simulink model "prestudio55"  (R2018b)
settings: Solver=ode45  StartTime=0.  StopTime=20  FixedStep=0.2  MaxStep=0.05  RelTol=1e-8  AbsTol=1e-8  EnableMultiTasking=on
settings Model: ExtModeTrigMode=oneshot  ExtModeArmWhenConnect=off  Creator=LEVIENKL  LastModifiedBy=Heidi Reed
settings SolverCC: AutoScaleAbsTol=off
settings DataIOCC: SaveFormat=Array  SignalLoggingSaveFormat=ModelDataLogs  SaveOutput=off  SaveTime=off  SignalLoggingName=sigsOut
settings OptimizationCC: BlockReduction=off  BooleanDataType=off  ExpressionDepthLimit=2147483647  InitFltsAndDblsToZero=on  LifeSpan=inf
settings DebuggingCC: SaveWithParameterizedLinksMsg=none  UnderspecifiedInitializationDetection=Classic  MergeDetectMultiDrivingBlocksExec=none  SignalResolutionControl=TryResolveAllWithWarning  MultiTaskDSMMsg=warning  MultiTaskCondExecSysMsg=none  FcnCallInpInsideContextMsg=warning  AllowSymbolicDim=off  StateNameClashWarn=warning  SFUnexpectedBacktrackingDiag=warning  SFNoUnconditionalDefaultTransitionDiag=warning  SFExecutionAtInitializationDiag=none
settings HardwareCC: ProdBitPerPointer=32  ProdBitPerSizeT=32  ProdBitPerPtrDiffT=32  ProdLargestAtomicFloat=None  ProdIntDivRoundTo=Undefined  ProdEndianess=Unspecified  ProdWordSize=32  ProdHWDeviceType=32-bit Generic  TargetUnknown=on
settings ModelReferenceCC: PropagateSignalLabelsOutOfModel=off
settings SFSimCC: SimUseLocalCustomCode=off
settings RTWCC: RTWUseLocalCustomCode=off
settings CodeAppCC: StateflowObjectComments=on
settings GRTTargetCC: TargetFcnLib=ansi_tfl_tmw.mat  TargetLangStandard=C89/C90 (ANSI)  CombineOutputUpdateFcns=off  GRTInterface=on
settings ConfigComp: CovMetricSettings=dw  CovHtmlReporting=on  CovSaveCumulativeToWorkspaceVar=on  CovSaveSingleToWorkspaceVar=on  CovExternalEMLEnable=off  CovSFcnEnable=off

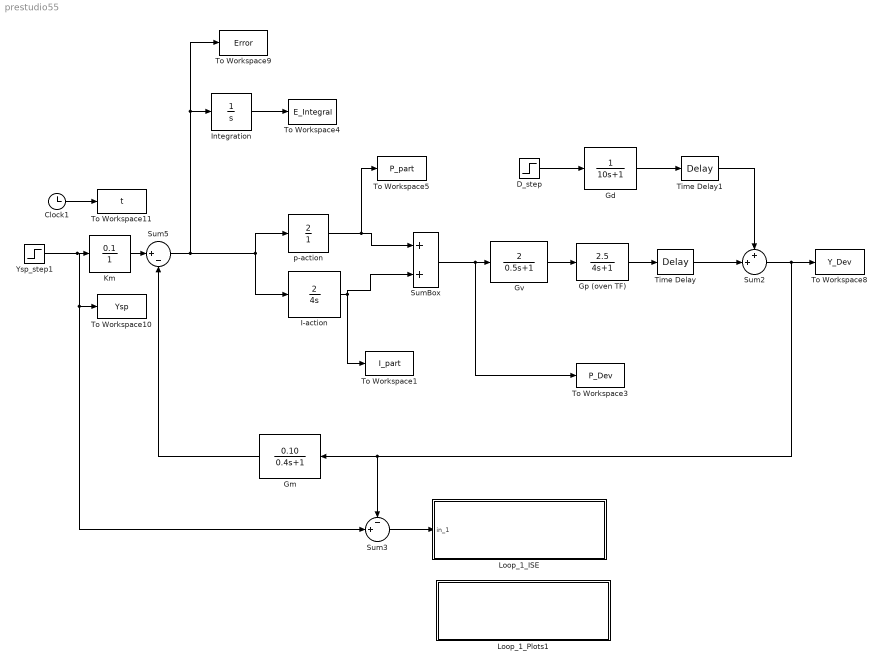
== system prestudio55 ==
  Clock1 : Clock
  D_step : Step  Time=0  After=0  SampleTime=0
      settings: AttributesFormatString=%<Before> to %<After>\nat %<Time>
  Gd : TransferFcn  Denominator=[10 1]
  Gm : TransferFcn  Numerator=[0.10]  Denominator=[0.4 1]
  Gp (oven TF) : TransferFcn  Numerator=[2.5]  Denominator=[4 1]
  Gv : TransferFcn  Numerator=[2]  Denominator=[0.5 1]
  "I-action " : TransferFcn  Numerator=[2]  Denominator=[4 0]
  "Integration " : TransferFcn  Denominator=[1 0]
  "Km " : TransferFcn  Numerator=[0.1]  Denominator=[0 1]
  Loop_1_ISE : Subsystem  mask(Integral Squarred Evaluation - Loop 1){}
      settings: OpenFcn=ISE1
      mask Help: This block calculates and plots loop #1 ISE.
      mask Display: disp('After Loop 1 Simulation:\n Double Click for ISE evaluation\n (uses ISE1.p)')
  Loop_1_Plots1 : Subsystem  mask(Y,U,E Plots - Loop 1){}
      settings: OpenFcn=YPEplots
      mask Help: This block loop #1 Y,U,Error in 3x1 Figure Window.
      mask Display: disp('After Loop 1 Simulation:\n Double Click for Y, P, Error Plots\n (uses YPEplots.p)')
  Sum2 : Sum  Inputs=++|  InputSameDT=on  SaturateOnIntegerOverflow=on  OutDataTypeStr=Inherit: Same as first input
  Sum3 : Sum  Inputs=-+|  InputSameDT=on  SaturateOnIntegerOverflow=on  OutDataTypeStr=Inherit: Same as first input
  Sum5 : Sum  Inputs=|+-  InputSameDT=on  SaturateOnIntegerOverflow=on  OutDataTypeStr=Inherit: Same as first input
  SumBox : Sum
  Time Delay : TransportDelay  DelayTime=0
      settings: AttributesFormatString=Delay=%<DelayTime>
  Time Delay1 : TransportDelay  DelayTime=0
      settings: AttributesFormatString=Delay=%<DelayTime>
  To Workspace1 : ToWorkspace  VariableName=I_part  SampleTime=-1
  To Workspace10 : ToWorkspace  VariableName=Ysp  SampleTime=-1
  To Workspace11 : ToWorkspace  VariableName=t  SampleTime=-1
  To Workspace3 : ToWorkspace  VariableName=P_Dev  SampleTime=-1
  To Workspace4 : ToWorkspace  VariableName=E_Integral  SampleTime=-1
  To Workspace5 : ToWorkspace  VariableName=P_part  SampleTime=-1
  To Workspace8 : ToWorkspace  VariableName=Y_Dev  SampleTime=-1
  To Workspace9 : ToWorkspace  VariableName=Error  SampleTime=-1
  Ysp_step1 : Step  Time=2  After=5  SampleTime=0
      settings: AttributesFormatString=%<Before> to %<After>\nat %<Time>
  "p-action " : TransferFcn  Numerator=[2]  Denominator=[0 1]
  wires:
  Ysp_step1/1 -> "Km "/1, Sum3/2, To Workspace10/1
  Sum5/1 -> "p-action "/1, "I-action "/1, "Integration "/1, To Workspace9/1
  "I-action "/1 -> SumBox/2, To Workspace1/1
  "p-action "/1 -> To Workspace5/1, SumBox/1
  SumBox/1 -> Gv/1, To Workspace3/1
  "Km "/1 -> Sum5/1
  Clock1/1 -> To Workspace11/1
  Sum3/1 -> Loop_1_ISE/1(in_1)
  Gm/1 -> Sum5/2
  Gv/1 -> Gp (oven TF)/1
  "Integration "/1 -> To Workspace4/1
  D_step/1 -> Gd/1
  Gd/1 -> Time Delay1/1
  Time Delay1/1 -> Sum2/1
  Gp (oven TF)/1 -> Time Delay/1
  Time Delay/1 -> Sum2/2
  Sum2/1 -> Gm/1, Sum3/1, To Workspace8/1

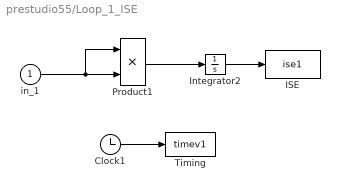
== system prestudio55/Loop_1_ISE ==
  in_1 : Inport
  Clock1 : Clock
  ISE : ToWorkspace  VariableName=ise1
      settings: MaxDataPoints=20000
  Integrator2 : Integrator
  Product1 : Product  InputSameDT=on  RndMeth=Zero  SaturateOnIntegerOverflow=on  OutDataTypeStr=Inherit: Same as first input
  Timing : ToWorkspace  VariableName=timev1
      settings: MaxDataPoints=20000
  wires:
  in_1/1 -> Product1/2, Product1/1
  Integrator2/1 -> ISE/1
  Clock1/1 -> Timing/1
  Product1/1 -> Integrator2/1

== system prestudio55/Loop_1_Plots1 ==
